simulink model "HDVPSG_DelayComp_NewRef_RealDrop_case1"  (R2019b)
settings: Solver=FixedStepDiscrete  StartTime=0.0  StopTime=28  FixedStep=UT.Ts_Veh  RelTol=1e-3
PostLoadFcn:
  | if any(exist('dsrtsu_mdlpostloadfcn', 'file') ~= 0), dsrtsu_mdlpostloadfcn('Execute', bdroot); end
InitFcn:
  | , if any(exist('dsmpb_private', 'file') ~= 0), dsmpb_private('dsmpb_mdlclblib', 'Init', bdroot); end,
values from neighbouring files (symbols this model uses):
  BETA_HDV_Leader = 50    [HDVPSG_DelayComp_NewRef_RealDrop_script_case1.m]
  BETA_PSG_Follower = 150    [HDVPSG_DelayComp_NewRef_RealDrop_script_case1.m]
  CtrlZone_Length = 250    [HDVPSG_DelayComp_NewRef_RealDrop_script_case1.m]
  DELTA_D_MIN = 5    [HDVPSG_DelayComp_NewRef_RealDrop_script_case1.m]
  DELTA_DR_MG_TCC = 15    [HDVPSG_DelayComp_NewRef_RealDrop_script_case1.m]
  HDV_AMAX = 1.3    [HDVPSG_DelayComp_NewRef_RealDrop_script_case1.m]
  HDV_AMIN = -2.5    [HDVPSG_DelayComp_NewRef_RealDrop_script_case1.m]
  HDV_first_v0 = 13    [HDVPSG_DelayComp_NewRef_RealDrop_script_case1.m]
  HDV_HighMu_D = 9    [HDVPSG_DelayComp_NewRef_RealDrop_script_case1.m]
  HDV_HighMu_I = 27    [HDVPSG_DelayComp_NewRef_RealDrop_script_case1.m]
  HDV_HighMu_P = 27    [HDVPSG_DelayComp_NewRef_RealDrop_script_case1.m]
  HDV_HighMu_TRFC = 0.7    [HDVPSG_DelayComp_NewRef_RealDrop_script_case1.m]
  HDV_last_v0 = 13    [HDVPSG_DelayComp_NewRef_RealDrop_script_case1.m]
  HDV_LowMu_D = 6    [HDVPSG_DelayComp_NewRef_RealDrop_script_case1.m]
  HDV_LowMu_I = 8    [HDVPSG_DelayComp_NewRef_RealDrop_script_case1.m]
  HDV_LowMu_P = 12    [HDVPSG_DelayComp_NewRef_RealDrop_script_case1.m]
  HDV_LowMu_TRFC = 0.6    [HDVPSG_DelayComp_NewRef_RealDrop_script_case1.m]
  Np_MPC = 20    [HDVPSG_DelayComp_NewRef_RealDrop_script_case1.m]
  PSG_AMAX = 3.2    [HDVPSG_DelayComp_NewRef_RealDrop_script_case1.m]
  PSG_AMIN = -6    [HDVPSG_DelayComp_NewRef_RealDrop_script_case1.m]
  PSG_end_v0 = 13    [HDVPSG_DelayComp_NewRef_RealDrop_script_case1.m]
  PSG_first_v0 = 13    [HDVPSG_DelayComp_NewRef_RealDrop_script_case1.m]
  PSG_HighMu_D = 15    [HDVPSG_DelayComp_NewRef_RealDrop_script_case1.m]
  PSG_HighMu_I = 125    [HDVPSG_DelayComp_NewRef_RealDrop_script_case1.m]
  PSG_HighMu_P = 75    [HDVPSG_DelayComp_NewRef_RealDrop_script_case1.m]
  PSG_HighMu_TRFC = 0.8    [HDVPSG_DelayComp_NewRef_RealDrop_script_case1.m]
  PSG_LowMu_D = 12    [HDVPSG_DelayComp_NewRef_RealDrop_script_case1.m]
  PSG_LowMu_I = 64    [HDVPSG_DelayComp_NewRef_RealDrop_script_case1.m]
  PSG_LowMu_P = 48    [HDVPSG_DelayComp_NewRef_RealDrop_script_case1.m]
  PSG_LowMu_TRFC = 0.7    [HDVPSG_DelayComp_NewRef_RealDrop_script_case1.m]
  PSG_middle_v0 = 13    [HDVPSG_DelayComp_NewRef_RealDrop_script_case1.m]
  Q_Leader = 1    [HDVPSG_DelayComp_NewRef_RealDrop_script_case1.m]
  Qd_dot_PSG_Follower = 2    [HDVPSG_DelayComp_NewRef_RealDrop_script_case1.m]
  Qd_PSG_Follower = 10    [HDVPSG_DelayComp_NewRef_RealDrop_script_case1.m]
  R_Leader = 20    [HDVPSG_DelayComp_NewRef_RealDrop_script_case1.m]
  R_PSG_Follower = 1    [HDVPSG_DelayComp_NewRef_RealDrop_script_case1.m]
  Recved_40_1 = Recved_Flag_Combined(47740,:)    [HDVPSG_DelayComp_NewRef_RealDrop_script_case1.m]
  Recved_40_2 = Recved_Flag_Combined(47780,:)    [HDVPSG_DelayComp_NewRef_RealDrop_script_case1.m]
  Recved_40_3 = Recved_Flag_Combined(49536,:)    [HDVPSG_DelayComp_NewRef_RealDrop_script_case1.m]
  Recved_40_4 = Recved_Flag_Combined(118106,:)    [HDVPSG_DelayComp_NewRef_RealDrop_script_case1.m]
  Rho_deltad_PSG_Follower = 1e3    (= 1000)    [HDVPSG_DelayComp_NewRef_RealDrop_script_case1.m]
  Rho_v_PSG_Follower = 1e3    (= 1000)    [HDVPSG_DelayComp_NewRef_RealDrop_script_case1.m]
  T_ADE = 0.01    [HDVPSG_DelayComp_NewRef_RealDrop_script_case1.m]
  V_MAX = 40    [HDVPSG_DelayComp_NewRef_RealDrop_script_case1.m]
  V_MIN = 0    [HDVPSG_DelayComp_NewRef_RealDrop_script_case1.m]
  VR_MG_TCC = 15    [HDVPSG_DelayComp_NewRef_RealDrop_script_case1.m]
undefined symbols (not defined in the file or in its folder): DiscIntNeverNeededParam, UT
libraries: simulink x46
(part 2 of 16)

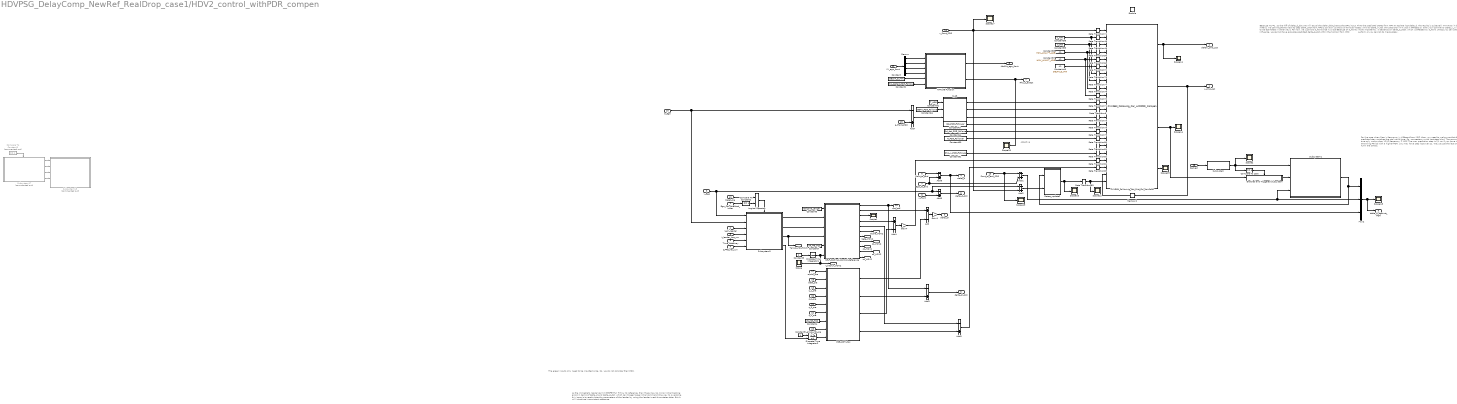
== system HDVPSG_DelayComp_NewRef_RealDrop_case1/HDV2_control_withPDR_compen ==
  note: The green inputs only need to be inputted once. So, we do not consider their PDR.
  note: Use the predicted states from MPC to replace lost delta_d, the results is quitewell;
      |
      | However, it does not work for delta_d_dot, the prediciton of d_dot is affected by both your command (delta_v_r), but more importantly, it depends on delta_d_ddot, which is affected by a_front. Unless you can predict a_front, or you cannot do it accurately.
  note: Because Hc =1, so the diff of delta_d_dot_pre will equal the delta_ddot_hat as the MPC input.
      | That means, we cannot get the next Np step delta_ddot from MPC's solution; so the a of front car needs to be estimated in other ways.
      | For now, we just hold a_front once it is lost
      |
      | Because of a_front's influence, we cannot have accurate predicted delta_d_dot within the horizon from MPC
  note: Adaptive
  note: For the case when Recv's frequency is different from MPC, then you need to make sure that the predicted step matches the real world time. So, we create a novel Lost-step block
      |
      | The commented one only works when V2VC freqeucny = MPC
      |
      | The max prediction step is 21, so if you have Large Sampling Period with a higher PDR, you may have step lost over 21. We just use the last one to fulfill the others.
  note: As the immediate leader cannot PERFECTLY follow its reference, then there may be minor initial tracking errors in terms of delta_d and delta_d_dot, which can trigger large initial command
      |
      | One way to overcome this issue is to recalculate the parameters of the leader by using the leader's real-time states data. But it will introduce inconsistant reference
  Ego_CtrL_enabled_Index : Inport
  t_all_leader : Inport  Port=2
  t_leader_has_run : Inport  Port=3
  t_PRE_has_run : Inport  Port=4
  Time_headway : Inport  Port=5
  Front_to_end : Inport  Port=6
  Ego_to_end : Inport  Port=7
  v_Front : Inport  Port=8
  v_Ego : Inport  Port=9
  a_Ego : Inport  Port=10
  XY_ego_front : Inport  Port=11
  Reset_sig : Inport  Port=12
  Front_to_end_PDR : Inport  Port=13
  v_Front_PDR : Inport  Port=14
  a_Front_PDR : Inport  Port=15
  Recved : Inport  Port=16
  alpha_pre : Inport  Port=17
  beta_pre : Inport  Port=18
  c_1_pre : Inport  Port=19
  c_2_pre : Inport  Port=20
  c_3_pre : Inport  Port=21
  c_4_pre : Inport  Port=22
  T_all_to_MP_pre : Inport  Port=23
  Enable : EnablePort
  Add : Sum  Inputs=+-
  Add{1..3,5..8} (7 alike) : Sum  Inputs=-+
  Add4 : Sum  Inputs=+-
  CVXGEN_Following_Car_Dist_Ctrl_NonSoft2 : S-Function  Description=Simulink:masks:SFunctionBuilder_MD  InitFcn=try, set_param(gcb,'FunctionName','CVXGEN_Following_Car_withPDR_Compen'), end  FunctionName=CVXGEN_Following_Car_withPDR_Compen  SFunctionModules=CVXGEN_Following_Car_withPDR_Compen_wrapper solver util matrix_support ldl  SFunctionDeploymentMode=off  EnableBusSupport=off
      mask init:
      | val = [[.9  0.75 0.75 1 1 .9 .9 1]',[1 1 0.75 0.75 .9 .9 1 .9]'];try , sys = get_param(gcb,'SfunBuilderFcnName');if isempty(sys), sys = get_param(gcb,'FunctionName'); end,catch, sys = get_param(gcb,'FunctionName'); end
      settings: CopyFcn=set_param(gcbh,'LinkStatus','none')  PreSaveFcn=try, set_param(gcb,'FunctionName','CVXGEN_Following_Car_withPDR_Compen'), end  OpenFcn=sfunctionwizard(gcbh)
      mask Display: plot(val(:,1),val(:,2)),disp(sys), port_label('input',1,'v_front_car'), port_label('input',2,'vmax'), port_label('input',3,'vmin'), port_label('input',4,'deltav_max'), port_label('input',5,'deltav_min'), port_label('input',6,'deltad_min'), port_label('input',7,'vcmd_max'), port_label('input',8,'vcmd_min'), port_label('input',9,'delta_vcmd_max'), port_label('input',10,'delta_vcmd_min'), port_label('input',11,'A'), port_label('input',12,'B'), port_label('input',13,'d_k'), port_label('input',14,'Q_deltad'), port_label('input',15,'Q_deltad_dot'), port_label('input',16,'R'), port_label('input',17,'Rho_deltad'), port_label('input',18,'Rho_v'), port_label('input',19,'deltad_r'), port_label('input',20,'deltad_dot_r'), port_label('input',21,'v_cmd_last'), port_label('input',22,'x_0'), port_label('output',1,'delta_v_cmd_opt'), port_label('output',2,'v_cmd_opt'), port_label('output',3,'delta_d_pre'), port_label('output',4,'delta_d_dot_pre')
  Compare To Constant2 : simulink/Logic and Bit Operations/Compare To Constant  relop===  const=1  OutDataTypeStr=boolean
  Compare To Constant3 : simulink/Logic and Bit Operations/Compare To Constant  Commented=on  relop===  const=1  OutDataTypeStr=boolean
  Compare To Zero : simulink/Logic and Bit Operations/Compare To Zero  relop===  OutDataTypeStr=boolean
  Constant : Constant  Value=DELTA_D_MIN
  Constant2 : Constant  Value=Rho_deltad_PSG_Follower
  Constant3 : Constant
  Constant4 : Constant  Value=VR_MG_TCC
  Constant42 : Constant  Value=T_ADE
  Constant43 : Constant  Value=Qd_PSG_Follower
  Constant44 : Constant  Value=Qd_dot_PSG_Follower
  Constant45 : Constant  Value=DELTA_D_MIN
  Constant5 : Constant
  Constant50 : Constant  Value=R_PSG_Follower
  Constant51 : Constant  Value=Rho_v_PSG_Follower
  Constant55 : Constant  Value=HDV_AMAX*T_ADE
  Constant57 : Constant  Value=HDV_AMIN*T_ADE
  Constant58 : Constant  Value=V_MAX
  Constant59 : Constant  Value=V_MIN
  Constant6 : Constant  Value=CtrlZone_Length
  Constant61 : Constant  Value=BETA_PSG_Follower
  Constant7 : Constant  Value=VR_MG_TCC
  Demux : Demux
  Discrete-Time Integrator1 : DiscreteIntegrator  SampleTime=-1  ICPrevOutput=DiscIntNeverNeededParam  ICPrevScaledInput=DiscIntNeverNeededParam
  Discrete-Time Integrator2 : DiscreteIntegrator  InitialConditionSource=external  SampleTime=-1  ICPrevOutput=DiscIntNeverNeededParam  ICPrevScaledInput=DiscIntNeverNeededParam
  Enabled and Triggered Subsystem : Subsystem  TreatAsAtomicUnit=on
  Gain1 : Gain  Gain=-1
  Gain4 : Gain  Gain=-1
  Logical Operator : Logic  Operator=OR  AllPortsSameDT=off  OutDataTypeStr=boolean
  MATLAB Function : MATLAB Function  TreatAsAtomicUnit=on
  Memory2 : Memory  InitialCondition=PSG_end_v0
  Mux2 : Mux  Inputs=3
  PRE_OPT_Pos : MATLAB Function  TreatAsAtomicUnit=on
  Rate Transition{6,48..50,68,70..85} (21 alike) : RateTransition
  SELF_Optimal_Control_Reference : MATLAB Function  TreatAsAtomicUnit=on
  Scope{,1..2,10..12,14..19} (12 alike) : Scope
  States_update2 : MATLAB Function  TreatAsAtomicUnit=on
  Subsystem : Subsystem
  Subsystem1 : Subsystem
  Subsystem17 : Subsystem  Commented=on
  Subsystem18 : Subsystem  Commented=on
  Subsystem3 : Subsystem
  Sys3 : MATLAB Function  TreatAsAtomicUnit=on
  v_cmd_opt : Outport
  deltav_cmd_opt : Outport  Port=2
  delta_dr : Outport  Port=3
  delta_d : Outport  Port=4
  delta_dr_dot : Outport  Port=5
  delta_d_dot : Outport  Port=6
  Rho_d_adapt : Outport  Port=7
  AbsDis_ego_front : Outport  Port=8
  delta_d_against_PDR : Outport  Port=9
  opt_spd : Outport  Port=10
  alpha_HDV2 : Outport  Port=11
  beta_HDV2 : Outport  Port=12
  c1_HDV2 : Outport  Port=13
  c2_HDV2 : Outport  Port=14
  c3_HDV2 : Outport  Port=15
  c4_HDV2 : Outport  Port=16
  Tall_to_MP_HDV2 : Outport  Port=17
  t_hasrun_HDV2 : Outport  Port=18
  wires:
  Add2/1 -> States_update2/2(delta_d_dot)
  Front_to_end/1 -> Add8/1
  Mux2/1 -> Scope18/1, delta_d_against_PDR/1
  Enabled and Triggered Subsystem/1(delta_d_pre_freeze) -> Subsystem1/2(delta_d_pre_freeze_if_lost)
  Compare To Zero/1 -> Enabled and Triggered Subsystem/Enable
  CVXGEN_Following_Car_Dist_Ctrl_NonSoft2/4 -> Scope15/1
  CVXGEN_Following_Car_Dist_Ctrl_NonSoft2/3 -> Enabled and Triggered Subsystem/1(delta_d_pre), Scope14/1
  Recved/1 -> Subsystem/1(Recv)
  MATLAB Function/1(REALWORLD_DIST) -> AbsDis_ego_front/1
  Compare To Constant3/1 -> Subsystem17/Enable
  Subsystem17/2(a_1) -> Subsystem18/2(a1)
  Subsystem17/4(a_3) -> Subsystem18/4(a3)
  Subsystem17/3(a_2) -> Subsystem18/3(a2)
  Subsystem17/1(a_0) -> Subsystem18/1(a0)
  Constant2/1 -> MATLAB Function/6(Rho_delta_dMAX)
  Constant/1 -> MATLAB Function/5(DELTA_D_MIN)
  Demux/4 -> MATLAB Function/4(Y_Front)  "Y_front"
  Demux/3 -> MATLAB Function/3(X_Front)  "X_front"
  Demux/2 -> MATLAB Function/2(Y_Ego)  "Y_ego"
  Demux/1 -> MATLAB Function/1(X_Ego)  "X_ego"
  XY_ego_front/1 -> Demux/1
  t_all_leader/1 -> Subsystem3/3(t_all_leader)
  Add6/1 -> delta_d_dot/1
  Rate Transition72/1 -> CVXGEN_Following_Car_Dist_Ctrl_NonSoft2/6
  Rate Transition75/1 -> CVXGEN_Following_Car_Dist_Ctrl_NonSoft2/14
  Rate Transition76/1 -> CVXGEN_Following_Car_Dist_Ctrl_NonSoft2/7
  Rate Transition78/1 -> CVXGEN_Following_Car_Dist_Ctrl_NonSoft2/9
  Rate Transition50/1 -> CVXGEN_Following_Car_Dist_Ctrl_NonSoft2/4
  States_update2/1(x0) -> Rate Transition83/1, Scope16/1
  Rate Transition80/1 -> CVXGEN_Following_Car_Dist_Ctrl_NonSoft2/16
  Constant45/1 -> Rate Transition72/1
  Sys3/1(A) -> Rate Transition71/1
  Rate Transition48/1 -> CVXGEN_Following_Car_Dist_Ctrl_NonSoft2/2
  Ego_CtrL_enabled_Index/1 -> Compare To Constant2/1
  Add7/1 -> Sys3/3(delta_d_ddot_hat)
  Rate Transition74/1 -> CVXGEN_Following_Car_Dist_Ctrl_NonSoft2/1
  Add8/1 -> delta_d/1, Mux2/3
  Memory2/1 -> CVXGEN_Following_Car_Dist_Ctrl_NonSoft2/21
  Rate Transition6/1 -> CVXGEN_Following_Car_Dist_Ctrl_NonSoft2/12
  Sys3/2(B) -> Rate Transition6/1
  Rate Transition49/1 -> CVXGEN_Following_Car_Dist_Ctrl_NonSoft2/3
  Rate Transition85/1 -> CVXGEN_Following_Car_Dist_Ctrl_NonSoft2/20
  MATLAB Function/2(Rho_delta_d_adpt) -> Scope10/1, Rho_d_adapt/1
  Constant61/1 -> Sys3/2(beta)
  Rate Transition81/1 -> CVXGEN_Following_Car_Dist_Ctrl_NonSoft2/17
  CVXGEN_Following_Car_Dist_Ctrl_NonSoft2/2 -> Memory2/1, v_cmd_opt/1  "v_cmd_opt"
  Constant50/1 -> Rate Transition80/1
  Constant43/1 -> Rate Transition75/1
  Rate Transition82/1 -> CVXGEN_Following_Car_Dist_Ctrl_NonSoft2/18
  Rate Transition71/1 -> CVXGEN_Following_Car_Dist_Ctrl_NonSoft2/11
  Rate Transition84/1 -> CVXGEN_Following_Car_Dist_Ctrl_NonSoft2/19
  Sys3/3(dk) -> Rate Transition73/1
  Constant42/1 -> Sys3/1(Ts)
  Constant44/1 -> Rate Transition79/1
  Constant55/1 -> Rate Transition50/1, Rate Transition78/1
  Rate Transition77/1 -> CVXGEN_Following_Car_Dist_Ctrl_NonSoft2/8
  Constant58/1 -> Rate Transition48/1, Rate Transition76/1
  v_Ego/1 -> Add2/1, Add6/1, Subsystem3/1(v_ego)
  Rate Transition79/1 -> CVXGEN_Following_Car_Dist_Ctrl_NonSoft2/15
  v_Front/1 -> Add6/2
  CVXGEN_Following_Car_Dist_Ctrl_NonSoft2/1 -> Scope11/1, deltav_cmd_opt/1
  Constant59/1 -> Rate Transition49/1, Rate Transition77/1
  Rate Transition70/1 -> CVXGEN_Following_Car_Dist_Ctrl_NonSoft2/10
  Rate Transition68/1 -> CVXGEN_Following_Car_Dist_Ctrl_NonSoft2/5
  Constant51/1 -> Rate Transition82/1
  Ego_to_end/1 -> Add8/2, Add1/2
  a_Ego/1 -> Subsystem3/2(a_ego), Add7/1  "a_ego"
  Rate Transition83/1 -> Scope12/1, CVXGEN_Following_Car_Dist_Ctrl_NonSoft2/22
  Rate Transition73/1 -> CVXGEN_Following_Car_Dist_Ctrl_NonSoft2/13
  Constant57/1 -> Rate Transition68/1, Rate Transition70/1
  Time_headway/1 -> Subsystem3/5(Time_headway)
  t_leader_has_run/1 -> Subsystem3/4(t_leader_has_run)
  Compare To Constant2/1 -> Logical Operator/2
  Logical Operator/1 -> Subsystem3/Enable
  Reset_sig/1 -> Logical Operator/1
  Add1/1 -> Subsystem1/3(delta_d_measure), Mux2/2
  Front_to_end_PDR/1 -> Add1/1, Scope19/1
  v_Front_PDR/1 -> Add2/2, Rate Transition74/1, Scope17/1
  a_Front_PDR/1 -> Add7/2
  Constant3/1 -> Discrete-Time Integrator1/1
  Discrete-Time Integrator1/1 -> Scope/1, t_hasrun_HDV2/1, SELF_Optimal_Control_Reference/6(t_aft_trigger)
  Constant7/1 -> SELF_Optimal_Control_Reference/5(v_mp)
  Constant6/1 -> SELF_Optimal_Control_Reference/1(L_ctz)
  Subsystem3/1(v_ego_ini) -> SELF_Optimal_Control_Reference/2(v_ini)
  Subsystem3/2(a_ego_ini) -> SELF_Optimal_Control_Reference/3(a_ini)
  Subsystem3/3(T_all_to_MP_ego) -> SELF_Optimal_Control_Reference/4(T_all_to_MP), Tall_to_MP_HDV2/1
  SELF_Optimal_Control_Reference/1(opt_spd) -> Add3/1, opt_spd/1
  SELF_Optimal_Control_Reference/2(opt_pos) -> Add/1
  alpha_pre/1 -> PRE_OPT_Pos/1(alpha_pre)
  beta_pre/1 -> PRE_OPT_Pos/2(beta_pre)
  c_1_pre/1 -> PRE_OPT_Pos/3(c_1_pre)
  c_2_pre/1 -> PRE_OPT_Pos/4(c_2_pre)
  c_3_pre/1 -> PRE_OPT_Pos/5(c_3_pre)
  c_4_pre/1 -> PRE_OPT_Pos/6(c_4_pre)
  Constant4/1 -> PRE_OPT_Pos/7(v_mp)
  Discrete-Time Integrator2/1 -> PRE_OPT_Pos/9(t_aft_trigger_pre)
  Constant5/1 -> Discrete-Time Integrator2/1
  t_PRE_has_run/1 -> Subsystem3/6(t_PRE_has_run)
  Subsystem3/4(t_PRE_has_run_ini) -> Discrete-Time Integrator2/2
  T_all_to_MP_pre/1 -> PRE_OPT_Pos/8(T_all_to_MP_pre)
  PRE_OPT_Pos/1(opt_pos_pre) -> Add/2
  Add/1 -> Gain1/1
  PRE_OPT_Pos/2(opt_spd_pre) -> Add3/2
  Add3/1 -> delta_dr_dot/1
  Add4/1 -> Gain4/1
  SELF_Optimal_Control_Reference/4(opt_pos_vec) -> Add4/1
  PRE_OPT_Pos/3(opt_pos_pre_vec) -> Add4/2
  PRE_OPT_Pos/4(opt_spd_pre_vec) -> Add5/2
  SELF_Optimal_Control_Reference/5(opt_spd_vec) -> Add5/1
  Add5/1 -> Rate Transition85/1
  Gain1/1 -> delta_dr/1
  Gain4/1 -> Rate Transition84/1
  SELF_Optimal_Control_Reference/3(opt_acc) -> Scope1/1
  SELF_Optimal_Control_Reference/6(alpha) -> alpha_HDV2/1
  SELF_Optimal_Control_Reference/7(beta) -> beta_HDV2/1
  SELF_Optimal_Control_Reference/8(c_1) -> c1_HDV2/1
  SELF_Optimal_Control_Reference/9(c_2) -> c2_HDV2/1
  SELF_Optimal_Control_Reference/10(c_3) -> c3_HDV2/1
  SELF_Optimal_Control_Reference/11(c_4) -> c4_HDV2/1
  Subsystem1/1(delta_d_enhanced) -> States_update2/1(delta_d), Mux2/1
  Subsystem/1(Lost_Step) -> Scope2/1, Subsystem1/1(Lost_Step), Compare To Zero/1

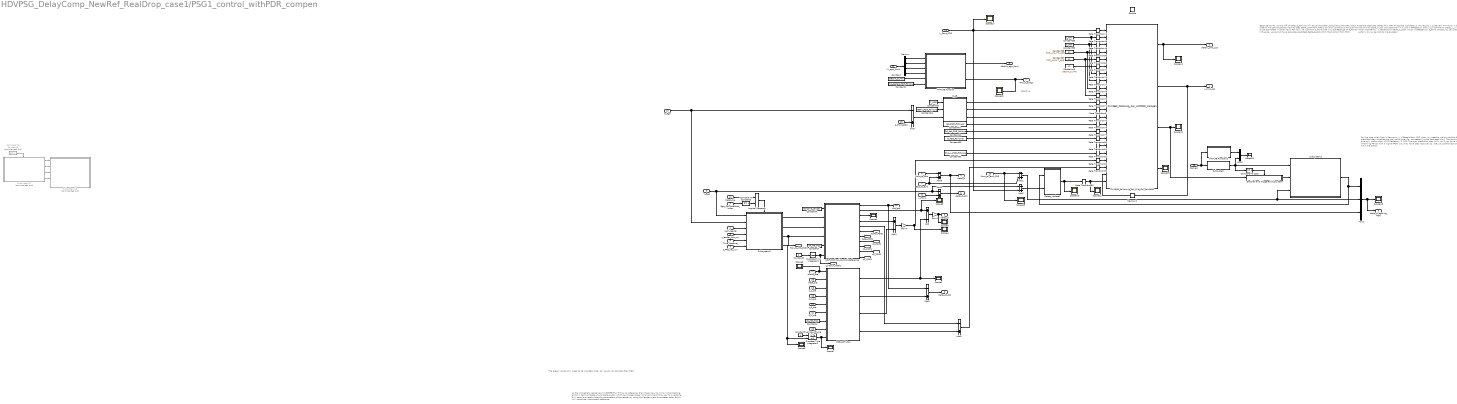
== system HDVPSG_DelayComp_NewRef_RealDrop_case1/PSG1_control_withPDR_compen ==
  note: As the immediate leader cannot PERFECTLY follow its reference, then there may be minor initial tracking errors in terms of delta_d and delta_d_dot, which can trigger large initial command
      |
      | One way to overcome this issue is to recalculate the parameters of the leader by using the leader's real-time states data. But it will introduce inconsistant reference
  note: For the case when Recv's frequency is different from MPC, then you need to make sure that the predicted step matches the real world time. So, we create a novel Lost-step block
      |
      | The commented one only works when V2VC freqeucny = MPC
      |
      | The max prediction step is 21, so if you have Large Sampling Period with a higher PDR, you may have step lost over 21. We just use the last one to fulfill the others.
  note: Adaptive
  note: Because Hc =1, so the diff of delta_d_dot_pre will equal the delta_ddot_hat as the MPC input.
      | That means, we cannot get the next Np step delta_ddot from MPC's solution; so the a of front car needs to be estimated in other ways.
      | For now, we just hold a_front once it is lost
      |
      | Because of a_front's influence, we cannot have accurate predicted delta_d_dot within the horizon from MPC
  note: Use the predicted states from MPC to replace lost delta_d, the results is quitewell;
      |
      | However, it does not work for delta_d_dot, the prediciton of d_dot is affected by both your command (delta_v_r), but more importantly, it depends on delta_d_ddot, which is affected by a_front. Unless you can predict a_front, or you cannot do it accurately.
  note: The green inputs only need to be inputted once. So, we do not consider their PDR.
  Ego_CtrL_enabled_Index : Inport
  t_all_leader : Inport  Port=2
  t_leader_has_run : Inport  Port=3
  t_PRE_has_run : Inport  Port=4
  Time_headway : Inport  Port=5
  Front_to_end : Inport  Port=6
  Ego_to_end : Inport  Port=7
  v_Front : Inport  Port=8
  v_Ego : Inport  Port=9
  a_Ego : Inport  Port=10
  XY_ego_front : Inport  Port=11
  Reset_sig : Inport  Port=12
  Front_to_end_PDR : Inport  Port=13
  v_Front_PDR : Inport  Port=14
  a_Front_PDR : Inport  Port=15
  Recved : Inport  Port=16
  alpha_pre : Inport  Port=17
  beta_pre : Inport  Port=18
  c_1_pre : Inport  Port=19
  c_2_pre : Inport  Port=20
  c_3_pre : Inport  Port=21
  c_4_pre : Inport  Port=22
  T_all_to_MP_pre : Inport  Port=23
  Enable : EnablePort
  Add : Sum  Inputs=+-
  Add{1..3,5..8} (7 alike) : Sum  Inputs=-+
  Add4 : Sum  Inputs=+-
  CVXGEN_Following_Car_Dist_Ctrl_NonSoft2 : S-Function  Description=Simulink:masks:SFunctionBuilder_MD  InitFcn=try, set_param(gcb,'FunctionName','CVXGEN_Following_Car_withPDR_Compen'), end  FunctionName=CVXGEN_Following_Car_withPDR_Compen  SFunctionModules=CVXGEN_Following_Car_withPDR_Compen_wrapper solver util matrix_support ldl  SFunctionDeploymentMode=off  EnableBusSupport=off
      mask init: same as HDVPSG_DelayComp_NewRef_RealDrop_case1/HDV2_control_withPDR_compen/CVXGEN_Following_Car_Dist_Ctrl_NonSoft2
      settings: CopyFcn=set_param(gcbh,'LinkStatus','none')  PreSaveFcn=try, set_param(gcb,'FunctionName','CVXGEN_Following_Car_withPDR_Compen'), end  OpenFcn=sfunctionwizard(gcbh)
      mask Display: plot(val(:,1),val(:,2)),disp(sys), port_label('input',1,'v_front_car'), port_label('input',2,'vmax'), port_label('input',3,'vmin'), port_label('input',4,'deltav_max'), port_label('input',5,'deltav_min'), port_label('input',6,'deltad_min'), port_label('input',7,'vcmd_max'), port_label('input',8,'vcmd_min'), port_label('input',9,'delta_vcmd_max'), port_label('input',10,'delta_vcmd_min'), port_label('input',11,'A'), port_label('input',12,'B'), port_label('input',13,'d_k'), port_label('input',14,'Q_deltad'), port_label('input',15,'Q_deltad_dot'), port_label('input',16,'R'), port_label('input',17,'Rho_deltad'), port_label('input',18,'Rho_v'), port_label('input',19,'deltad_r'), port_label('input',20,'deltad_dot_r'), port_label('input',21,'v_cmd_last'), port_label('input',22,'x_0'), port_label('output',1,'delta_v_cmd_opt'), port_label('output',2,'v_cmd_opt'), port_label('output',3,'delta_d_pre'), port_label('output',4,'delta_d_dot_pre')
  Compare To Constant2 : simulink/Logic and Bit Operations/Compare To Constant  relop===  const=1  OutDataTypeStr=boolean
  Compare To Constant3 : simulink/Logic and Bit Operations/Compare To Constant  Commented=on  relop===  const=1  OutDataTypeStr=boolean
  Compare To Zero : simulink/Logic and Bit Operations/Compare To Zero  relop===  OutDataTypeStr=boolean
  Constant : Constant  Value=DELTA_D_MIN
  Constant2 : Constant  Value=Rho_deltad_PSG_Follower
  Constant3 : Constant
  Constant4 : Constant  Value=VR_MG_TCC
  Constant42 : Constant  Value=T_ADE
  Constant43 : Constant  Value=Qd_PSG_Follower
  Constant44 : Constant  Value=Qd_dot_PSG_Follower
  Constant45 : Constant  Value=DELTA_D_MIN
  Constant5 : Constant
  Constant50 : Constant  Value=R_PSG_Follower
  Constant51 : Constant  Value=Rho_v_PSG_Follower
  Constant55 : Constant  Value=PSG_AMAX*T_ADE
  Constant57 : Constant  Value=PSG_AMIN*T_ADE
  Constant58 : Constant  Value=V_MAX
  Constant59 : Constant  Value=V_MIN
  Constant6 : Constant  Value=CtrlZone_Length
  Constant61 : Constant  Value=BETA_PSG_Follower
  Constant7 : Constant  Value=VR_MG_TCC
  Demux : Demux
  Discrete-Time Integrator1 : DiscreteIntegrator  SampleTime=-1  ICPrevOutput=DiscIntNeverNeededParam  ICPrevScaledInput=DiscIntNeverNeededParam
  Discrete-Time Integrator2 : DiscreteIntegrator  InitialConditionSource=external  SampleTime=-1  ICPrevOutput=DiscIntNeverNeededParam  ICPrevScaledInput=DiscIntNeverNeededParam
  Enabled and Triggered Subsystem : Subsystem  TreatAsAtomicUnit=on
  Gain1 : Gain  Gain=-1
  Gain4 : Gain  Gain=-1
  Logical Operator : Logic  Operator=OR  AllPortsSameDT=off  OutDataTypeStr=boolean
  MATLAB Function : MATLAB Function  TreatAsAtomicUnit=on
  MATLAB Function2 : MATLAB Function  TreatAsAtomicUnit=on
  Memory2 : Memory  InitialCondition=PSG_end_v0
  Mux2 : Mux  Inputs=3
  Mux3 : Mux  Inputs=2
  PRE_OPT_Pos : MATLAB Function  TreatAsAtomicUnit=on
  Rate Transition{6,48..50,68,70..85} (21 alike) : RateTransition
  SELF_Optimal_Control_Reference : MATLAB Function  TreatAsAtomicUnit=on
  Scope{1..8,10..12,14..19,21} (18 alike) : Scope
  States_update2 : MATLAB Function  TreatAsAtomicUnit=on
  Subsystem : Subsystem
  Subsystem17 : Subsystem  Commented=on
  Subsystem18 : Subsystem  Commented=on
  Subsystem2 : Subsystem
  Subsystem3 : Subsystem
  Sys3 : MATLAB Function  TreatAsAtomicUnit=on
  v_cmd_opt : Outport
  deltav_cmd_opt : Outport  Port=2
  delta_dr : Outport  Port=3
  delta_d : Outport  Port=4
  delta_dr_dot : Outport  Port=5
  delta_d_dot : Outport  Port=6
  Rho_d_adapt : Outport  Port=7
  AbsDis_ego_front : Outport  Port=8
  delta_d_against_PDR : Outport  Port=9
  opt_spd : Outport  Port=10
  alpha_PSG1 : Outport  Port=11
  beta_PSG1 : Outport  Port=12
  c1_PSG1 : Outport  Port=13
  c2_PSG1 : Outport  Port=14
  c3_PSG1 : Outport  Port=15
  c4_PSG1 : Outport  Port=16
  Tall_to_MP_PSG1 : Outport  Port=17
  t_hasrun_PSG1 : Outport  Port=18
  wires:
  SELF_Optimal_Control_Reference/11(c_4) -> c4_PSG1/1
  SELF_Optimal_Control_Reference/10(c_3) -> c3_PSG1/1
  SELF_Optimal_Control_Reference/9(c_2) -> c2_PSG1/1
  SELF_Optimal_Control_Reference/8(c_1) -> c1_PSG1/1
  SELF_Optimal_Control_Reference/7(beta) -> beta_PSG1/1
  SELF_Optimal_Control_Reference/6(alpha) -> alpha_PSG1/1
  SELF_Optimal_Control_Reference/3(opt_acc) -> Scope1/1
  Gain4/1 -> Scope4/1, Rate Transition84/1
  Gain1/1 -> Scope5/1, delta_dr/1
  Add5/1 -> Rate Transition85/1
  SELF_Optimal_Control_Reference/5(opt_spd_vec) -> Add5/1
  PRE_OPT_Pos/4(opt_spd_pre_vec) -> Add5/2
  PRE_OPT_Pos/3(opt_pos_pre_vec) -> Add4/2
  SELF_Optimal_Control_Reference/4(opt_pos_vec) -> Add4/1
  Add4/1 -> Gain4/1
  Add3/1 -> delta_dr_dot/1
  PRE_OPT_Pos/2(opt_spd_pre) -> Add3/2
  Add/1 -> Gain1/1
  PRE_OPT_Pos/1(opt_pos_pre) -> Scope2/1, Add/2
  T_all_to_MP_pre/1 -> PRE_OPT_Pos/8(T_all_to_MP_pre)
  Subsystem3/4(t_PRE_has_run_ini) -> Scope8/1, Discrete-Time Integrator2/2
  t_PRE_has_run/1 -> Subsystem3/6(t_PRE_has_run)
  Constant5/1 -> Discrete-Time Integrator2/1
  Discrete-Time Integrator2/1 -> Scope7/1, PRE_OPT_Pos/9(t_aft_trigger_pre)
  Constant4/1 -> PRE_OPT_Pos/7(v_mp)
  c_4_pre/1 -> PRE_OPT_Pos/6(c_4_pre)
  c_3_pre/1 -> PRE_OPT_Pos/5(c_3_pre)
  c_2_pre/1 -> PRE_OPT_Pos/4(c_2_pre)
  c_1_pre/1 -> PRE_OPT_Pos/3(c_1_pre)
  beta_pre/1 -> PRE_OPT_Pos/2(beta_pre)
  alpha_pre/1 -> Scope6/1, PRE_OPT_Pos/1(alpha_pre)
  SELF_Optimal_Control_Reference/2(opt_pos) -> Scope3/1, Add/1
  SELF_Optimal_Control_Reference/1(opt_spd) -> opt_spd/1, Add3/1
  Subsystem3/3(T_all_to_MP_ego) -> Tall_to_MP_PSG1/1, SELF_Optimal_Control_Reference/4(T_all_to_MP)
  Subsystem3/2(a_ego_ini) -> SELF_Optimal_Control_Reference/3(a_ini)
  Subsystem3/1(v_ego_ini) -> SELF_Optimal_Control_Reference/2(v_ini)
  Constant6/1 -> SELF_Optimal_Control_Reference/1(L_ctz)
  Constant7/1 -> SELF_Optimal_Control_Reference/5(v_mp)
  Discrete-Time Integrator1/1 -> SELF_Optimal_Control_Reference/6(t_aft_trigger), t_hasrun_PSG1/1
  Constant3/1 -> Discrete-Time Integrator1/1
  Subsystem/1(Lost_Step) -> Subsystem2/1(Lost_Step), Compare To Zero/1, Mux3/2
  Mux3/1 -> Scope21/1
  MATLAB Function2/1(Lost_Step) -> Mux3/1
  a_Front_PDR/1 -> Add7/2
  v_Front_PDR/1 -> Scope17/1, Rate Transition74/1, Add2/2
  Front_to_end_PDR/1 -> Scope19/1, Add1/1
  Add1/1 -> Subsystem2/3(delta_d_measure), Mux2/2
  Reset_sig/1 -> Logical Operator/1
  Logical Operator/1 -> Subsystem3/Enable
  Compare To Constant2/1 -> Logical Operator/2
  t_leader_has_run/1 -> Subsystem3/4(t_leader_has_run)
  Time_headway/1 -> Subsystem3/5(Time_headway)
  Constant57/1 -> Rate Transition70/1, Rate Transition68/1
  Rate Transition73/1 -> CVXGEN_Following_Car_Dist_Ctrl_NonSoft2/13
  Rate Transition83/1 -> CVXGEN_Following_Car_Dist_Ctrl_NonSoft2/22, Scope12/1
  a_Ego/1 -> Add7/1, Subsystem3/2(a_ego)  "a_ego"
  Ego_to_end/1 -> Add1/2, Add8/2
  Constant51/1 -> Rate Transition82/1
  Rate Transition68/1 -> CVXGEN_Following_Car_Dist_Ctrl_NonSoft2/5
  Rate Transition70/1 -> CVXGEN_Following_Car_Dist_Ctrl_NonSoft2/10
  Constant59/1 -> Rate Transition77/1, Rate Transition49/1
  CVXGEN_Following_Car_Dist_Ctrl_NonSoft2/1 -> deltav_cmd_opt/1, Scope11/1
  v_Front/1 -> Add6/2
  Rate Transition79/1 -> CVXGEN_Following_Car_Dist_Ctrl_NonSoft2/15
  v_Ego/1 -> Subsystem3/1(v_ego), Add6/1, Add2/1
  Constant58/1 -> Rate Transition76/1, Rate Transition48/1
  Rate Transition77/1 -> CVXGEN_Following_Car_Dist_Ctrl_NonSoft2/8
  Constant55/1 -> Rate Transition78/1, Rate Transition50/1
  Constant44/1 -> Rate Transition79/1
  Constant42/1 -> Sys3/1(Ts)
  Sys3/3(dk) -> Rate Transition73/1
  Rate Transition84/1 -> CVXGEN_Following_Car_Dist_Ctrl_NonSoft2/19
  Rate Transition71/1 -> CVXGEN_Following_Car_Dist_Ctrl_NonSoft2/11
  Rate Transition82/1 -> CVXGEN_Following_Car_Dist_Ctrl_NonSoft2/18
  Constant43/1 -> Rate Transition75/1
  Constant50/1 -> Rate Transition80/1
  CVXGEN_Following_Car_Dist_Ctrl_NonSoft2/2 -> v_cmd_opt/1, Memory2/1  "v_cmd_opt"
  Rate Transition81/1 -> CVXGEN_Following_Car_Dist_Ctrl_NonSoft2/17
  Constant61/1 -> Sys3/2(beta)
  MATLAB Function/2(Rho_delta_d_adpt) -> Rho_d_adapt/1, Scope10/1
  Rate Transition85/1 -> CVXGEN_Following_Car_Dist_Ctrl_NonSoft2/20
  Rate Transition49/1 -> CVXGEN_Following_Car_Dist_Ctrl_NonSoft2/3
  Sys3/2(B) -> Rate Transition6/1
  Rate Transition6/1 -> CVXGEN_Following_Car_Dist_Ctrl_NonSoft2/12
  Memory2/1 -> CVXGEN_Following_Car_Dist_Ctrl_NonSoft2/21
  Add8/1 -> Mux2/3, delta_d/1
  Rate Transition74/1 -> CVXGEN_Following_Car_Dist_Ctrl_NonSoft2/1
  Add7/1 -> Sys3/3(delta_d_ddot_hat)
  Ego_CtrL_enabled_Index/1 -> Compare To Constant2/1
  Rate Transition48/1 -> CVXGEN_Following_Car_Dist_Ctrl_NonSoft2/2
  Sys3/1(A) -> Rate Transition71/1
  Constant45/1 -> Rate Transition72/1
  Rate Transition80/1 -> CVXGEN_Following_Car_Dist_Ctrl_NonSoft2/16
  States_update2/1(x0) -> Scope16/1, Rate Transition83/1
  Rate Transition50/1 -> CVXGEN_Following_Car_Dist_Ctrl_NonSoft2/4
  Rate Transition78/1 -> CVXGEN_Following_Car_Dist_Ctrl_NonSoft2/9
  Rate Transition76/1 -> CVXGEN_Following_Car_Dist_Ctrl_NonSoft2/7
  Rate Transition75/1 -> CVXGEN_Following_Car_Dist_Ctrl_NonSoft2/14
  Rate Transition72/1 -> CVXGEN_Following_Car_Dist_Ctrl_NonSoft2/6
  Add6/1 -> delta_d_dot/1
  t_all_leader/1 -> Subsystem3/3(t_all_leader)
  XY_ego_front/1 -> Demux/1
  Demux/1 -> MATLAB Function/1(X_Ego)  "X_ego"
  Demux/2 -> MATLAB Function/2(Y_Ego)  "Y_ego"
  Demux/3 -> MATLAB Function/3(X_Front)  "X_front"
  Demux/4 -> MATLAB Function/4(Y_Front)  "Y_front"
  Constant/1 -> MATLAB Function/5(DELTA_D_MIN)
  Constant2/1 -> MATLAB Function/6(Rho_delta_dMAX)
  Subsystem17/1(a_0) -> Subsystem18/1(a0)
  Subsystem17/3(a_2) -> Subsystem18/3(a2)
  Subsystem17/4(a_3) -> Subsystem18/4(a3)
  Subsystem17/2(a_1) -> Subsystem18/2(a1)
  Compare To Constant3/1 -> Subsystem17/Enable
  MATLAB Function/1(REALWORLD_DIST) -> AbsDis_ego_front/1
  Recved/1 -> MATLAB Function2/1(Recv), Subsystem/1(Recv)
  CVXGEN_Following_Car_Dist_Ctrl_NonSoft2/3 -> Scope14/1, Enabled and Triggered Subsystem/1(delta_d_pre)
  CVXGEN_Following_Car_Dist_Ctrl_NonSoft2/4 -> Scope15/1
  Compare To Zero/1 -> Enabled and Triggered Subsystem/Enable
  Enabled and Triggered Subsystem/1(delta_d_pre_freeze) -> Subsystem2/2(delta_d_pre_freeze_if_lost)
  Subsystem2/1(delta_d_enhanced) -> Mux2/1, States_update2/1(delta_d)
  Mux2/1 -> delta_d_against_PDR/1, Scope18/1
  Front_to_end/1 -> Add8/1
  Add2/1 -> States_update2/2(delta_d_dot)

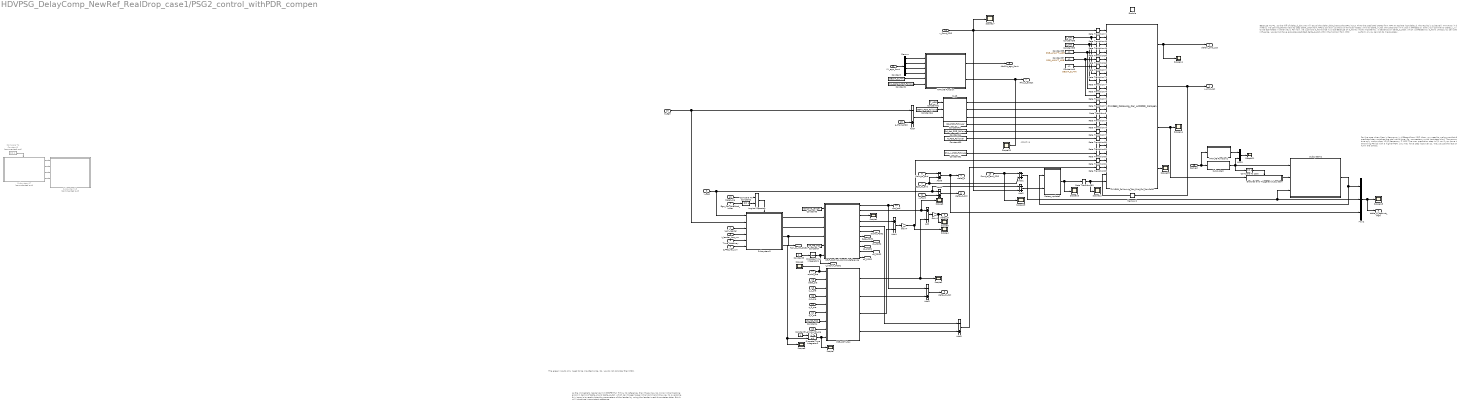
== system HDVPSG_DelayComp_NewRef_RealDrop_case1/PSG2_control_withPDR_compen ==
  note: The green inputs only need to be inputted once. So, we do not consider their PDR.
  note: Use the predicted states from MPC to replace lost delta_d, the results is quitewell;
      |
      | However, it does not work for delta_d_dot, the prediciton of d_dot is affected by both your command (delta_v_r), but more importantly, it depends on delta_d_ddot, which is affected by a_front. Unless you can predict a_front, or you cannot do it accurately.
  note: Because Hc =1, so the diff of delta_d_dot_pre will equal the delta_ddot_hat as the MPC input.
      | That means, we cannot get the next Np step delta_ddot from MPC's solution; so the a of front car needs to be estimated in other ways.
      | For now, we just hold a_front once it is lost
      |
      | Because of a_front's influence, we cannot have accurate predicted delta_d_dot within the horizon from MPC
  note: Adaptive
  note: For the case when Recv's frequency is different from MPC, then you need to make sure that the predicted step matches the real world time. So, we create a novel Lost-step block
      |
      | The commented one only works when V2VC freqeucny = MPC
      |
      | The max prediction step is 21, so if you have Large Sampling Period with a higher PDR, you may have step lost over 21. We just use the last one to fulfill the others.
  note: As the immediate leader cannot PERFECTLY follow its reference, then there may be minor initial tracking errors in terms of delta_d and delta_d_dot, which can trigger large initial command
      |
      | One way to overcome this issue is to recalculate the parameters of the leader by using the leader's real-time states data. But it will introduce inconsistant reference
  Ego_CtrL_enabled_Index : Inport
  t_all_leader : Inport  Port=2
  t_leader_has_run : Inport  Port=3
  t_PRE_has_run : Inport  Port=4
  Time_headway : Inport  Port=5
  Front_to_end : Inport  Port=6
  Ego_to_end : Inport  Port=7
  v_Front : Inport  Port=8
  v_Ego : Inport  Port=9
  a_Ego : Inport  Port=10
  XY_ego_front : Inport  Port=11
  Reset_sig : Inport  Port=12
  Front_to_end_PDR : Inport  Port=13
  v_Front_PDR : Inport  Port=14
  a_Front_PDR : Inport  Port=15
  Recved : Inport  Port=16
  alpha_pre : Inport  Port=17
  beta_pre : Inport  Port=18
  c_1_pre : Inport  Port=19
  c_2_pre : Inport  Port=20
  c_3_pre : Inport  Port=21
  c_4_pre : Inport  Port=22
  T_all_to_MP_pre : Inport  Port=23
  Enable : EnablePort
  Add : Sum  Inputs=+-
  Add{1..3,5..8} (7 alike) : Sum  Inputs=-+
  Add4 : Sum  Inputs=+-
  CVXGEN_Following_Car_Dist_Ctrl_NonSoft2 : S-Function  Description=Simulink:masks:SFunctionBuilder_MD  InitFcn=try, set_param(gcb,'FunctionName','CVXGEN_Following_Car_withPDR_Compen'), end  FunctionName=CVXGEN_Following_Car_withPDR_Compen  SFunctionModules=CVXGEN_Following_Car_withPDR_Compen_wrapper solver util matrix_support ldl  SFunctionDeploymentMode=off  EnableBusSupport=off
      mask init: same as HDVPSG_DelayComp_NewRef_RealDrop_case1/HDV2_control_withPDR_compen/CVXGEN_Following_Car_Dist_Ctrl_NonSoft2
      settings: CopyFcn=set_param(gcbh,'LinkStatus','none')  PreSaveFcn=try, set_param(gcb,'FunctionName','CVXGEN_Following_Car_withPDR_Compen'), end  OpenFcn=sfunctionwizard(gcbh)
      mask Display: plot(val(:,1),val(:,2)),disp(sys), port_label('input',1,'v_front_car'), port_label('input',2,'vmax'), port_label('input',3,'vmin'), port_label('input',4,'deltav_max'), port_label('input',5,'deltav_min'), port_label('input',6,'deltad_min'), port_label('input',7,'vcmd_max'), port_label('input',8,'vcmd_min'), port_label('input',9,'delta_vcmd_max'), port_label('input',10,'delta_vcmd_min'), port_label('input',11,'A'), port_label('input',12,'B'), port_label('input',13,'d_k'), port_label('input',14,'Q_deltad'), port_label('input',15,'Q_deltad_dot'), port_label('input',16,'R'), port_label('input',17,'Rho_deltad'), port_label('input',18,'Rho_v'), port_label('input',19,'deltad_r'), port_label('input',20,'deltad_dot_r'), port_label('input',21,'v_cmd_last'), port_label('input',22,'x_0'), port_label('output',1,'delta_v_cmd_opt'), port_label('output',2,'v_cmd_opt'), port_label('output',3,'delta_d_pre'), port_label('output',4,'delta_d_dot_pre')
  Compare To Constant2 : simulink/Logic and Bit Operations/Compare To Constant  relop===  const=1  OutDataTypeStr=boolean
  Compare To Constant3 : simulink/Logic and Bit Operations/Compare To Constant  Commented=on  relop===  const=1  OutDataTypeStr=boolean
  Compare To Zero : simulink/Logic and Bit Operations/Compare To Zero  relop===  OutDataTypeStr=boolean
  Constant : Constant  Value=DELTA_D_MIN
  Constant2 : Constant  Value=Rho_deltad_PSG_Follower
  Constant3 : Constant
  Constant4 : Constant  Value=VR_MG_TCC
  Constant42 : Constant  Value=T_ADE
  Constant43 : Constant  Value=Qd_PSG_Follower
  Constant44 : Constant  Value=Qd_dot_PSG_Follower
  Constant45 : Constant  Value=DELTA_D_MIN
  Constant5 : Constant
  Constant50 : Constant  Value=R_PSG_Follower
  Constant51 : Constant  Value=Rho_v_PSG_Follower
  Constant55 : Constant  Value=PSG_AMAX*T_ADE
  Constant57 : Constant  Value=PSG_AMIN*T_ADE
  Constant58 : Constant  Value=V_MAX
  Constant59 : Constant  Value=V_MIN
  Constant6 : Constant  Value=CtrlZone_Length
  Constant61 : Constant  Value=BETA_PSG_Follower
  Constant7 : Constant  Value=VR_MG_TCC
  Demux : Demux
  Discrete-Time Integrator1 : DiscreteIntegrator  SampleTime=-1  ICPrevOutput=DiscIntNeverNeededParam  ICPrevScaledInput=DiscIntNeverNeededParam
  Discrete-Time Integrator2 : DiscreteIntegrator  InitialConditionSource=external  SampleTime=-1  ICPrevOutput=DiscIntNeverNeededParam  ICPrevScaledInput=DiscIntNeverNeededParam
  Enabled and Triggered Subsystem : Subsystem  TreatAsAtomicUnit=on
  Gain1 : Gain  Gain=-1
  Gain4 : Gain  Gain=-1
  Logical Operator : Logic  Operator=OR  AllPortsSameDT=off  OutDataTypeStr=boolean
  MATLAB Function : MATLAB Function  TreatAsAtomicUnit=on
  MATLAB Function2 : MATLAB Function  TreatAsAtomicUnit=on
  Memory2 : Memory  InitialCondition=PSG_end_v0
  Mux2 : Mux  Inputs=3
  Mux3 : Mux  Inputs=2
  PRE_OPT_Pos : MATLAB Function  TreatAsAtomicUnit=on
  Rate Transition{6,48..50,68,70..85} (21 alike) : RateTransition
  SELF_Optimal_Control_Reference : MATLAB Function  TreatAsAtomicUnit=on
  Scope{1..8,10..12,14..19,21} (18 alike) : Scope
  States_update2 : MATLAB Function  TreatAsAtomicUnit=on
  Subsystem : Subsystem
  Subsystem17 : Subsystem  Commented=on
  Subsystem18 : Subsystem  Commented=on
  Subsystem2 : Subsystem
  Subsystem3 : Subsystem
  Sys3 : MATLAB Function  TreatAsAtomicUnit=on
  v_cmd_opt : Outport
  deltav_cmd_opt : Outport  Port=2
  delta_dr : Outport  Port=3
  delta_d : Outport  Port=4
  delta_dr_dot : Outport  Port=5
  delta_d_dot : Outport  Port=6
  Rho_d_adapt : Outport  Port=7
  AbsDis_ego_front : Outport  Port=8
  delta_d_against_PDR : Outport  Port=9
  opt_spd : Outport  Port=10
  alpha_PSG2 : Outport  Port=11
  beta_PSG2 : Outport  Port=12
  c1_PSG2 : Outport  Port=13
  c2_PSG2 : Outport  Port=14
  c3_PSG2 : Outport  Port=15
  c4_PSG2 : Outport  Port=16
  Tall_to_MP_PSG2 : Outport  Port=17
  t_hasrun_PSG2 : Outport  Port=18
  wires:
  Add2/1 -> States_update2/2(delta_d_dot)
  Front_to_end/1 -> Add8/1
  Mux2/1 -> Scope18/1, delta_d_against_PDR/1
  Subsystem2/1(delta_d_enhanced) -> States_update2/1(delta_d), Mux2/1
  Enabled and Triggered Subsystem/1(delta_d_pre_freeze) -> Subsystem2/2(delta_d_pre_freeze_if_lost)
  Compare To Zero/1 -> Enabled and Triggered Subsystem/Enable
  CVXGEN_Following_Car_Dist_Ctrl_NonSoft2/4 -> Scope15/1
  CVXGEN_Following_Car_Dist_Ctrl_NonSoft2/3 -> Enabled and Triggered Subsystem/1(delta_d_pre), Scope14/1
  Recved/1 -> Subsystem/1(Recv), MATLAB Function2/1(Recv)
  MATLAB Function/1(REALWORLD_DIST) -> AbsDis_ego_front/1
  Compare To Constant3/1 -> Subsystem17/Enable
  Subsystem17/2(a_1) -> Subsystem18/2(a1)
  Subsystem17/4(a_3) -> Subsystem18/4(a3)
  Subsystem17/3(a_2) -> Subsystem18/3(a2)
  Subsystem17/1(a_0) -> Subsystem18/1(a0)
  Constant2/1 -> MATLAB Function/6(Rho_delta_dMAX)
  Constant/1 -> MATLAB Function/5(DELTA_D_MIN)
  Demux/4 -> MATLAB Function/4(Y_Front)  "Y_front"
  Demux/3 -> MATLAB Function/3(X_Front)  "X_front"
  Demux/2 -> MATLAB Function/2(Y_Ego)  "Y_ego"
  Demux/1 -> MATLAB Function/1(X_Ego)  "X_ego"
  XY_ego_front/1 -> Demux/1
  t_all_leader/1 -> Subsystem3/3(t_all_leader)
  Add6/1 -> delta_d_dot/1
  Rate Transition72/1 -> CVXGEN_Following_Car_Dist_Ctrl_NonSoft2/6
  Rate Transition75/1 -> CVXGEN_Following_Car_Dist_Ctrl_NonSoft2/14
  Rate Transition76/1 -> CVXGEN_Following_Car_Dist_Ctrl_NonSoft2/7
  Rate Transition78/1 -> CVXGEN_Following_Car_Dist_Ctrl_NonSoft2/9
  Rate Transition50/1 -> CVXGEN_Following_Car_Dist_Ctrl_NonSoft2/4
  States_update2/1(x0) -> Rate Transition83/1, Scope16/1
  Rate Transition80/1 -> CVXGEN_Following_Car_Dist_Ctrl_NonSoft2/16
  Constant45/1 -> Rate Transition72/1
  Sys3/1(A) -> Rate Transition71/1
  Rate Transition48/1 -> CVXGEN_Following_Car_Dist_Ctrl_NonSoft2/2
  Ego_CtrL_enabled_Index/1 -> Compare To Constant2/1
  Add7/1 -> Sys3/3(delta_d_ddot_hat)
  Rate Transition74/1 -> CVXGEN_Following_Car_Dist_Ctrl_NonSoft2/1
  Add8/1 -> delta_d/1, Mux2/3
  Memory2/1 -> CVXGEN_Following_Car_Dist_Ctrl_NonSoft2/21
  Rate Transition6/1 -> CVXGEN_Following_Car_Dist_Ctrl_NonSoft2/12
  Sys3/2(B) -> Rate Transition6/1
  Rate Transition49/1 -> CVXGEN_Following_Car_Dist_Ctrl_NonSoft2/3
  Rate Transition85/1 -> CVXGEN_Following_Car_Dist_Ctrl_NonSoft2/20
  MATLAB Function/2(Rho_delta_d_adpt) -> Scope10/1, Rho_d_adapt/1
  Constant61/1 -> Sys3/2(beta)
  Rate Transition81/1 -> CVXGEN_Following_Car_Dist_Ctrl_NonSoft2/17
  CVXGEN_Following_Car_Dist_Ctrl_NonSoft2/2 -> Memory2/1, v_cmd_opt/1  "v_cmd_opt"
  Constant50/1 -> Rate Transition80/1
  Constant43/1 -> Rate Transition75/1
  Rate Transition82/1 -> CVXGEN_Following_Car_Dist_Ctrl_NonSoft2/18
  Rate Transition71/1 -> CVXGEN_Following_Car_Dist_Ctrl_NonSoft2/11
  Rate Transition84/1 -> CVXGEN_Following_Car_Dist_Ctrl_NonSoft2/19
  Sys3/3(dk) -> Rate Transition73/1
  Constant42/1 -> Sys3/1(Ts)
  Constant44/1 -> Rate Transition79/1
  Constant55/1 -> Rate Transition50/1, Rate Transition78/1
  Rate Transition77/1 -> CVXGEN_Following_Car_Dist_Ctrl_NonSoft2/8
  Constant58/1 -> Rate Transition48/1, Rate Transition76/1
  v_Ego/1 -> Add2/1, Add6/1, Subsystem3/1(v_ego)
  Rate Transition79/1 -> CVXGEN_Following_Car_Dist_Ctrl_NonSoft2/15
  v_Front/1 -> Add6/2
  CVXGEN_Following_Car_Dist_Ctrl_NonSoft2/1 -> Scope11/1, deltav_cmd_opt/1
  Constant59/1 -> Rate Transition49/1, Rate Transition77/1
  Rate Transition70/1 -> CVXGEN_Following_Car_Dist_Ctrl_NonSoft2/10
  Rate Transition68/1 -> CVXGEN_Following_Car_Dist_Ctrl_NonSoft2/5
  Constant51/1 -> Rate Transition82/1
  Ego_to_end/1 -> Add8/2, Add1/2
  a_Ego/1 -> Subsystem3/2(a_ego), Add7/1  "a_ego"
  Rate Transition83/1 -> Scope12/1, CVXGEN_Following_Car_Dist_Ctrl_NonSoft2/22
  Rate Transition73/1 -> CVXGEN_Following_Car_Dist_Ctrl_NonSoft2/13
  Constant57/1 -> Rate Transition68/1, Rate Transition70/1
  Time_headway/1 -> Subsystem3/5(Time_headway)
  t_leader_has_run/1 -> Subsystem3/4(t_leader_has_run)
  Compare To Constant2/1 -> Logical Operator/2
  Logical Operator/1 -> Subsystem3/Enable
  Reset_sig/1 -> Logical Operator/1
  Add1/1 -> Subsystem2/3(delta_d_measure), Mux2/2
  Front_to_end_PDR/1 -> Add1/1, Scope19/1
  v_Front_PDR/1 -> Add2/2, Rate Transition74/1, Scope17/1
  a_Front_PDR/1 -> Add7/2
  MATLAB Function2/1(Lost_Step) -> Mux3/1
  Mux3/1 -> Scope21/1
  Subsystem/1(Lost_Step) -> Subsystem2/1(Lost_Step), Mux3/2, Compare To Zero/1
  Constant3/1 -> Discrete-Time Integrator1/1
  Discrete-Time Integrator1/1 -> t_hasrun_PSG2/1, SELF_Optimal_Control_Reference/6(t_aft_trigger)
  Constant7/1 -> SELF_Optimal_Control_Reference/5(v_mp)
  Constant6/1 -> SELF_Optimal_Control_Reference/1(L_ctz)
  Subsystem3/1(v_ego_ini) -> SELF_Optimal_Control_Reference/2(v_ini)
  Subsystem3/2(a_ego_ini) -> SELF_Optimal_Control_Reference/3(a_ini)
  Subsystem3/3(T_all_to_MP_ego) -> SELF_Optimal_Control_Reference/4(T_all_to_MP), Tall_to_MP_PSG2/1
  SELF_Optimal_Control_Reference/1(opt_spd) -> Add3/1, opt_spd/1
  SELF_Optimal_Control_Reference/2(opt_pos) -> Add/1, Scope3/1
  alpha_pre/1 -> PRE_OPT_Pos/1(alpha_pre), Scope6/1
  beta_pre/1 -> PRE_OPT_Pos/2(beta_pre)
  c_1_pre/1 -> PRE_OPT_Pos/3(c_1_pre)
  c_2_pre/1 -> PRE_OPT_Pos/4(c_2_pre)
  c_3_pre/1 -> PRE_OPT_Pos/5(c_3_pre)
  c_4_pre/1 -> PRE_OPT_Pos/6(c_4_pre)
  Constant4/1 -> PRE_OPT_Pos/7(v_mp)
  Discrete-Time Integrator2/1 -> PRE_OPT_Pos/9(t_aft_trigger_pre), Scope7/1
  Constant5/1 -> Discrete-Time Integrator2/1
  t_PRE_has_run/1 -> Subsystem3/6(t_PRE_has_run)
  Subsystem3/4(t_PRE_has_run_ini) -> Discrete-Time Integrator2/2, Scope8/1
  T_all_to_MP_pre/1 -> PRE_OPT_Pos/8(T_all_to_MP_pre)
  PRE_OPT_Pos/1(opt_pos_pre) -> Add/2, Scope2/1
  Add/1 -> Gain1/1
  PRE_OPT_Pos/2(opt_spd_pre) -> Add3/2
  Add3/1 -> delta_dr_dot/1
  Add4/1 -> Gain4/1
  SELF_Optimal_Control_Reference/4(opt_pos_vec) -> Add4/1
  PRE_OPT_Pos/3(opt_pos_pre_vec) -> Add4/2
  PRE_OPT_Pos/4(opt_spd_pre_vec) -> Add5/2
  SELF_Optimal_Control_Reference/5(opt_spd_vec) -> Add5/1
  Add5/1 -> Rate Transition85/1
  Gain1/1 -> delta_dr/1, Scope5/1
  Gain4/1 -> Rate Transition84/1, Scope4/1
  SELF_Optimal_Control_Reference/3(opt_acc) -> Scope1/1
  SELF_Optimal_Control_Reference/6(alpha) -> alpha_PSG2/1
  SELF_Optimal_Control_Reference/7(beta) -> beta_PSG2/1
  SELF_Optimal_Control_Reference/8(c_1) -> c1_PSG2/1
  SELF_Optimal_Control_Reference/9(c_2) -> c2_PSG2/1
  SELF_Optimal_Control_Reference/10(c_3) -> c3_PSG2/1
  SELF_Optimal_Control_Reference/11(c_4) -> c4_PSG2/1
